simulink library "Springs_Axle2_None"  (R2026a)
settings: Solver=VariableStepAuto
libraries: fl_lib x4
Description:
  | Component of Simscape Vehicle Templates Library
  | 
  | Copyright 2018-2026 The MathWorks, Inc.
settings Model: Creator=smiller  LastModifiedBy=smiller

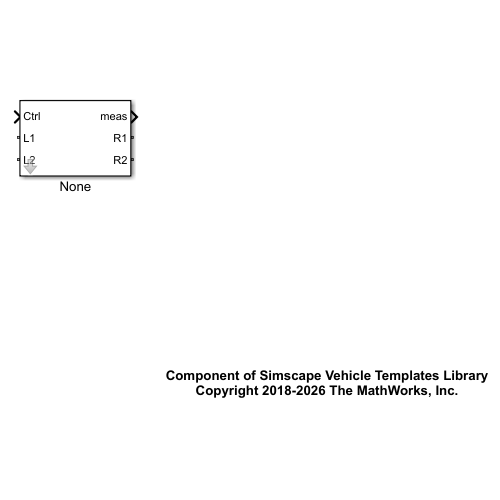
[thumbnail: Simulink's stored preview of the top-level diagram]
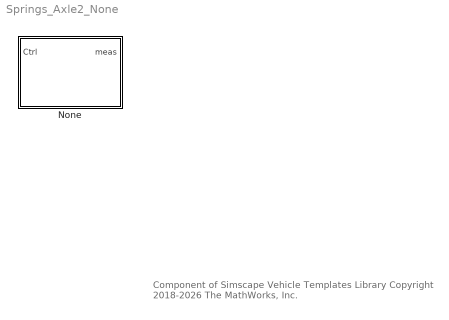
== system Springs_Axle2_None ==
  note: Component of Simscape Vehicle Templates Library
      | Copyright 2018-2026 The MathWorks, Inc.
  None : Subsystem  VariantControl=Independent  mask(Spring System Placeholder){InitTriggerDropdown=0}
      mask prompts: InitTriggerDropdown "Initialization Trigger Dropdown"
      mask help: Empty subsystem, used as a variant that omits springs.
      mask init:
      | curblk = gcb;
      | 
      | % Trigger Mask Initialization for 
      | % variant subsystems below this level
      | sm_car_lib_maskInitTrigger(curblk);
      mask TypeOptions InitTriggerDropdown: 0 | 1

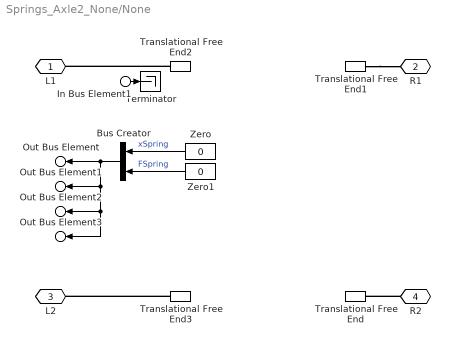
== system Springs_Axle2_None/None ==
  In Bus Element1 : Inport  PortName=Ctrl  Element=L1
  Bus Creator : BusCreator  Inputs=2
  Terminator : Terminator
  Translational Free End{,1..3} (4 alike) : fl_lib/Mechanical/Translational Elements/Translational Free End  v_specify=off  v_priority=None  v=0 m/s  v_nominal_specify=off  v_nominal_value=1  v_nominal_unit=m/s
  Zero : Constant  Value=0  OutDataTypeStr=Inherit: Inherit via back propagation
  Zero1 : Constant  Value=0  OutDataTypeStr=Inherit: Inherit via back propagation
  L1 : PMIOPort  Side=Left
  R1 : PMIOPort  Port=2  Side=Right
  L2 : PMIOPort  Port=3  Side=Left
  R2 : PMIOPort  Port=4  Side=Right
  Out Bus Element : Outport  VectorParamsAs1DForOutWhenUnconnected=off  PortName=meas  Element=L1
  Out Bus Element1 : Outport  VectorParamsAs1DForOutWhenUnconnected=off  PortName=meas  Element=R1
  Out Bus Element2 : Outport  VectorParamsAs1DForOutWhenUnconnected=off  PortName=meas  Element=L2
  Out Bus Element3 : Outport  VectorParamsAs1DForOutWhenUnconnected=off  PortName=meas  Element=R2
  wires:
  Bus Creator/1 -> Out Bus Element3/1, Out Bus Element2/1, Out Bus Element1/1, Out Bus Element/1
  In Bus Element1/1 -> Terminator/1
  Zero/1 -> Bus Creator/1  "xSpring"
  Zero1/1 -> Bus Creator/2  "FSpring"
  connections:
  Translational Free End2/LConn1 -- L1/RConn1
  Translational Free End3/LConn1 -- L2/RConn1
  R2/RConn1 -- Translational Free End/LConn1
  Translational Free End1/LConn1 -- R1/RConn1
